simulink model "Boat_sim"  (Simulink 7.8)
settings: Solver=FixedStepDiscrete  StartTime=0.0  StopTime=1000  FixedStep=.01  RelTol=1e-3
InitFcn:
  | clear all
  | missions
  | common
  | physical_constants
  | simulation_constants
  | initial_values
  | l2plus
values from neighbouring files (symbols this model uses):
  InitialPoint = 0    [l2plus.m]
  IPStar = 0    [l2plus.m]
  MaxDwnPthStar = 1    [l2plus.m]
  OC2max = 49999    [simulation_constants.m]
  phi_0 = 0    [simulation_constants.m]
  switchDistance = 4    [l2plus.m]
  T_step = 0.01    [common.m]
  tanIntercept = tan( 45*pi/180 )    [l2plus.m]
  TStar = single(4.5)    [l2plus.m]
  Turn2Track = 0    [l2plus.m]
  wheelbase = 3.27    [physical_constants.m]
undefined symbols (not defined in the file or in its folder): DiscIntNeverNeededParam, Earth, figure8_waypoints, sampling_waypoints, test_waypoints, WGS84
libraries: simulink x21, uSimLib x21, instrumentlib x2, aerolibtransform2 x1, aerolibanimutils x1, simulink_need_slupdate x1
(part 2 of 2)

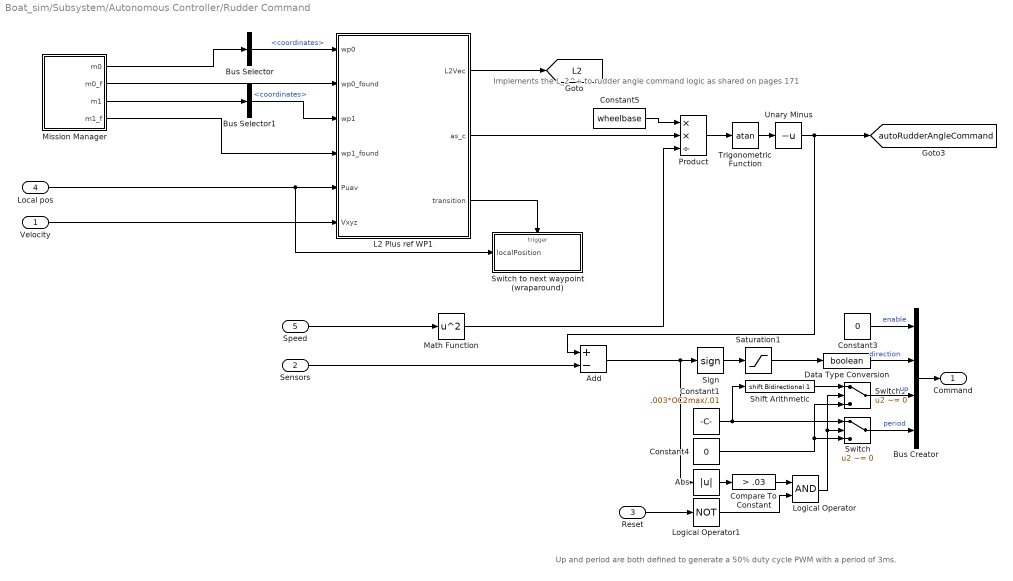
== system Boat_sim/Subsystem/Autonomous Controller/Rudder Command ==
  note: Up and period are both defined to generate a 50% duty cycle PWM with
      | a period of 3ms.
  note: Implements the L_2^+ to rudder angle command logic as shared on pages 171
  Velocity : Inport
  Sensors : Inport  Port=2
  Reset : Inport  Port=3
  Local pos : Inport  Port=4
  Speed : Inport  Port=5
  Abs : Abs
  Add : Sum  Inputs=+-
  Bus Creator : BusCreator
  Bus Selector : BusSelector  OutputSignals=coordinates
  Bus Selector1 : BusSelector  OutputSignals=coordinates
  Compare To Constant : simulink/Logic and Bit Operations/Compare To Constant  relop=>  const=.03  OutDataTypeStr=boolean
  Constant1 : Constant  Value=.003*OC2max/.01  OutDataTypeStr=uint16
  Constant3 : Constant  Value=0  OutDataTypeStr=boolean
  Constant4 : Constant  Value=0  OutDataTypeStr=uint16
  Constant5 : Constant  Value=wheelbase  OutDataTypeStr=boolean
  Data Type Conversion : DataTypeConversion  OutDataTypeStr=boolean  RndMeth=Simplest
  L2 Plus ref WP1 : MATLAB Function  TreatAsAtomicUnit=on
  Logical Operator : Logic  AllPortsSameDT=off  OutDataTypeStr=boolean
  Logical Operator1 : Logic  Operator=NOT  Inputs=1  AllPortsSameDT=off  OutDataTypeStr=boolean
  Math Function : Math  Operator=square  SaturateOnIntegerOverflow=on
  Mission Manager : Subsystem
  Product : Product  Inputs=**/  RndMeth=Zero
  Saturation1 : Saturate  UpperLimit=1  LowerLimit=0  OutDataTypeStr=Inherit: Inherit via back propagation
  Shift Arithmetic : ArithShift  BitShiftNumber=1
  Sign : Signum
  Switch : Switch  Criteria=u2 ~= 0
  Switch to next waypoint (wraparound) : Subsystem  TreatAsAtomicUnit=on
  Switch1 : Switch  Criteria=u2 ~= 0
  Trigonometric Function : Trigonometry  Operator=atan
  Unary Minus : UnaryMinus
  Command : Outport
  tag scope: L2=global, autoRudderAngleCommand=global
  wires:
  Bus Selector1/1 -> L2 Plus ref WP1/3(wp1)  "<coordinates>"
  Bus Selector/1 -> L2 Plus ref WP1/1(wp0)  "<coordinates>"
  Mission Manager/1(m0) -> Bus Selector/1
  Mission Manager/2(m0_f) -> L2 Plus ref WP1/2(wp0_found)
  L2 Plus ref WP1/3(transition) -> Switch to next waypoint (wraparound)/Trigger
  Mission Manager/4(m1_f) -> L2 Plus ref WP1/4(wp1_found)
  Mission Manager/3(m1) -> Bus Selector1/1
  Add/1 -> Abs/1, Sign/1
  Speed/1 -> Math Function/1
  Logical Operator1/1 -> Logical Operator/2
  Logical Operator/1 -> Switch1/2, Switch/2
  Compare To Constant/1 -> Logical Operator/1
  Local pos/1 -> Switch to next waypoint (wraparound)/1(localPosition), L2 Plus ref WP1/5(Puav)
  Reset/1 -> Logical Operator1/1
  Constant4/1 -> Switch1/3, Switch/3
  Switch1/1 -> Bus Creator/3  "up"
  Switch/1 -> Bus Creator/4  "period"
  Shift Arithmetic/1 -> Switch1/1
  Abs/1 -> Compare To Constant/1
  Constant1/1 -> Switch/1, Shift Arithmetic/1
  Constant3/1 -> Bus Creator/1  "enable"
  Velocity/1 -> L2 Plus ref WP1/6(Vxyz)
  L2 Plus ref WP1/1(L2Vec) -> [L2]
  Sign/1 -> Saturation1/1
  Saturation1/1 -> Data Type Conversion/1
  Bus Creator/1 -> Command/1
  Sensors/1 -> Add/2
  Data Type Conversion/1 -> Bus Creator/2  "direction"
  L2 Plus ref WP1/2(as_c) -> Product/2
  Constant5/1 -> Product/1
  Math Function/1 -> Product/3
  Product/1 -> Trigonometric Function/1
  Trigonometric Function/1 -> Unary Minus/1
  Unary Minus/1 -> Add/1, [autoRudderAngleCommand]

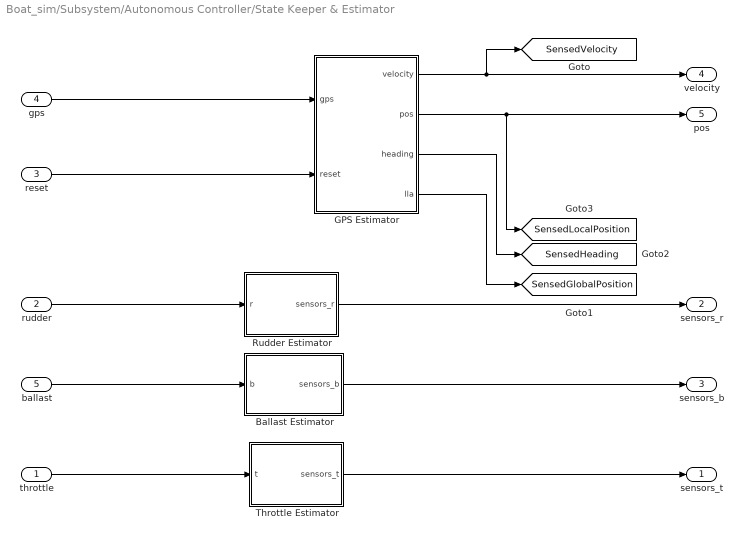
== system Boat_sim/Subsystem/Autonomous Controller/State Keeper & Estimator ==
  throttle : Inport
  rudder : Inport  Port=2
  reset : Inport  Port=3
  gps : Inport  Port=4
  ballast : Inport  Port=5
  Ballast Estimator : Subsystem
  GPS Estimator : Subsystem
  Rudder Estimator : Subsystem
  Throttle Estimator : Subsystem
  sensors_t : Outport
  sensors_r : Outport  Port=2
  sensors_b : Outport  Port=3
  velocity : Outport  Port=4
  pos : Outport  Port=5
  tag scope: SensedGlobalPosition=global, SensedHeading=global, SensedLocalPosition=global, SensedVelocity=global
  wires:
  Throttle Estimator/1(sensors_t) -> sensors_t/1
  Ballast Estimator/1(sensors_b) -> sensors_b/1
  Rudder Estimator/1(sensors_r) -> sensors_r/1
  GPS Estimator/4(lla) -> [SensedGlobalPosition]
  GPS Estimator/3(heading) -> [SensedHeading]
  GPS Estimator/2(pos) -> [SensedLocalPosition], pos/1
  gps/1 -> GPS Estimator/1(gps)
  GPS Estimator/1(velocity) -> [SensedVelocity], velocity/1
  reset/1 -> GPS Estimator/2(reset)
  throttle/1 -> Throttle Estimator/1(t)
  ballast/1 -> Ballast Estimator/1(b)
  rudder/1 -> Rudder Estimator/1(r)

== system Boat_sim/Subsystem/Autonomous Controller/Throttle Command ==
  sensors : Inport
  reset : Inport  Port=2
  Bus Creator : BusCreator
  Constant1 : Constant  Value=0  OutDataTypeStr=int16
  Constant5 : Constant  Value=1000  OutDataTypeStr=int16
  Mux Everything : Subsystem
  Switch : Switch  Criteria=u2 > Threshold
  Terminator : Terminator
  Trigger Events : Subsystem
  command : Outport
  tag scope: autoThrottleCommand=global
  wires:
  Constant5/1 -> Switch/3
  Constant1/1 -> Switch/1
  Switch/1 -> Trigger Events/1(RC Throttle), Mux Everything/4(Throttle), [autoThrottleCommand]
  Mux Everything/4(trig) -> Bus Creator/4  "trigger"
  Mux Everything/3(size) -> Bus Creator/3  "size"
  Mux Everything/2(data) -> Bus Creator/2  "data"
  Mux Everything/1(iden) -> Bus Creator/1  "identifier"
  reset/1 -> Switch/2, Trigger Events/2(Reset)
  Trigger Events/2(Disable) -> Mux Everything/2(disable)
  Trigger Events/3(Enable) -> Mux Everything/3(enable)
  Trigger Events/1(Change Speed) -> Mux Everything/1(speed)
  Bus Creator/1 -> command/1
  sensors/1 -> Terminator/1

== system Boat_sim/Subsystem/Log state data to workspace/Build HIL sentence ==
  data : Inport
  Bitwise Operator : simulink/Logic and Bit Operations/Bitwise Operator  logicop=XOR  UseBitMask=off  BitMask=bin2dec('11011001')  BitMaskRealWorld=Stored Integer
  Constant : Constant  Value=37  OutDataTypeStr=uint8
  Constant1 : Constant  Value=38  OutDataTypeStr=uint8
  Constant2 : Constant  Value=94  OutDataTypeStr=uint8
  Constant3 : Constant  Value=38  OutDataTypeStr=uint8
  Constant4 : Constant  Value=3  OutDataTypeStr=uint8
  Mux2 : Mux  Inputs=2
  Pack : MATLAB Function  TreatAsAtomicUnit=on
  sent : Outport
  wires:
  data/1 -> Mux2/2, Pack/4(d)
  Constant/1 -> Pack/1(a)
  Constant1/1 -> Pack/2(b)
  Pack/1(y) -> sent/1
  Constant4/1 -> Mux2/1, Pack/3(c)
  Constant2/1 -> Pack/5(e)
  Constant3/1 -> Pack/6(f)
  Bitwise Operator/1 -> Pack/7(g)
  Mux2/1 -> Bitwise Operator/1

== system Boat_sim/Plant/Actuator Dynamics/Subsystem/If Action Subsystem ==
  In1 : Inport
  Action Port : ActionPort  ActionType=then
  Bitwise Operator : simulink/Logic and Bit Operations/Bitwise Operator  logicop=OR  UseBitMask=off  NumInputPorts=2  BitMask=bin2dec('11011001')  BitMaskRealWorld=Stored Integer
  Data Store Write : DataStoreWrite  DataStoreName=throttle_speed
  Data Type Conversion : DataTypeConversion  OutDataTypeStr=uint16  ConvertRealWorld=Stored Integer (SI)
  Data Type Conversion2 : DataTypeConversion  OutDataTypeStr=double  LockScale=on
  Demux : Demux  Outputs=2
  Gain : Gain  Gain=1/1023
  Selector2 : Selector  InputPortWidth=6  IndexOptions=Index vector (dialog)  Indices=[4 3]  OutputSizes=1
  Shift Arithmetic : ArithShift  BitShiftNumber=-8
  wires:
  In1/1 -> Selector2/1
  Data Type Conversion2/1 -> Gain/1
  Gain/1 -> Data Store Write/1
  Selector2/1 -> Data Type Conversion/1
  Bitwise Operator/1 -> Data Type Conversion2/1
  Data Type Conversion/1 -> Demux/1
  Demux/1 -> Bitwise Operator/1
  Demux/2 -> Shift Arithmetic/1
  Shift Arithmetic/1 -> Bitwise Operator/2

== system Boat_sim/Subsystem/Autonomous Controller/Rudder Command/Mission Manager ==
  Data Type Conversion : DataTypeConversion  OutDataTypeStr=uint8
  GetCurrentMission : uSimLib/Mission Manager/GetCurrentMission  sampleTime=T_step
  GetMission : uSimLib/Mission Manager/GetMission  sampleTime=T_step
  If : If  IfExpression=u1 == 0
  If Action Subsystem : Subsystem  TreatAsAtomicUnit=on
  If Action Subsystem1 : Subsystem  TreatAsAtomicUnit=on
  Merge : Subsystem
  m0 : Outport
  m0_f : Outport  Port=2
  m1 : Outport  Port=3
  m1_f : Outport  Port=4
  wires:
  Data Type Conversion/1 -> GetMission/1
  Merge/2(found) -> m0_f/1
  Merge/1(mission) -> m0/1
  If Action Subsystem1/2(found) -> Merge/4(In4)
  If Action Subsystem/2(found) -> Merge/2(In3)
  If Action Subsystem1/1(mission) -> Merge/3(In2)
  If Action Subsystem/1(mission) -> Merge/1(In1)
  If/2 -> If Action Subsystem1/Action
  If/1 -> If Action Subsystem/Action
  GetMission/2 -> m1_f/1
  GetMission/1 -> m1/1
  GetCurrentMission/1 -> If/1, Data Type Conversion/1, If Action Subsystem1/1(i)

== system Boat_sim/Subsystem/Autonomous Controller/Rudder Command/Switch to next waypoint (wraparound) ==
  note: This block takes a triggering mission transition signal
      | and changes the current mission accordingly. It also
      | wraps the missions around if necessary from the last
      | mission to the first one.
  localPosition : Inport
  Trigger : TriggerPort
  Bias : Bias  Bias=1
  Data Type Conversion : DataTypeConversion  OutDataTypeStr=int8
  GetCurrentMission : uSimLib/Mission Manager/GetCurrentMission  sampleTime=-1
  GetMissionCount : uSimLib/Mission Manager/GetMissionCount  sampleTime=-1
  If : If  NumInputs=2  IfExpression=u1 < u2
  If Action Subsystem : Subsystem  TreatAsAtomicUnit=on
  If Action Subsystem1 : Subsystem  TreatAsAtomicUnit=on
  wires:
  localPosition/1 -> If Action Subsystem1/1(lPos)
  Data Type Conversion/1 -> If/2
  If/2 -> If Action Subsystem1/Action
  If/1 -> If Action Subsystem/Action
  Bias/1 -> If/1, If Action Subsystem/1(newIndex)
  GetMissionCount/1 -> Data Type Conversion/1
  GetCurrentMission/1 -> Bias/1

== system Boat_sim/Subsystem/Autonomous Controller/State Keeper & Estimator/Ballast Estimator ==
  b : Inport
  Bus Selector1 : BusSelector  OutputSignals=position
  sensors_b : Outport
  wires:
  Bus Selector1/1 -> sensors_b/1  "<position>"
  b/1 -> Bus Selector1/1

== system Boat_sim/Subsystem/Autonomous Controller/State Keeper & Estimator/GPS Estimator ==
  gps : Inport
  reset : Inport  Port=2
  Add : Sum
  Bus Selector1 : BusSelector  OutputSignals=newData
  Calculate local position from  GPS data : MATLAB Function  TreatAsAtomicUnit=on
  Discrete-Time Integrator4 : DiscreteIntegrator  ExternalReset=level  SampleTime=-1  ICPrevOutput=DiscIntNeverNeededParam  ICPrevScaledInput=DiscIntNeverNeededParam
  Subsystem : Subsystem
  velocity : Outport
  pos : Outport  Port=2
  heading : Outport  Port=3
  lla : Outport  Port=4
  tag scope: GpsOrigin=global, GpsOriginChanged=global
  wires:
  Calculate local position from  GPS data/4(refLLAChanged) -> [GpsOriginChanged]
  Calculate local position from  GPS data/3(refLLA) -> [GpsOrigin]
  Subsystem/1(velocity) -> Discrete-Time Integrator4/1, velocity/1
  Calculate local position from  GPS data/1(localPosition) -> Add/1
  Calculate local position from  GPS data/2(resetIntegrator) -> Discrete-Time Integrator4/2
  Bus Selector1/1 -> Calculate local position from  GPS data/2(newData)  "<newData>"
  Add/1 -> pos/1
  Discrete-Time Integrator4/1 -> Add/2
  Subsystem/3(pos) -> lla/1, Calculate local position from  GPS data/1(latLonAlt)
  gps/1 -> Bus Selector1/1, Subsystem/1(gps)
  Subsystem/2(heading) -> heading/1
  reset/1 -> Calculate local position from  GPS data/3(reset)

== system Boat_sim/Subsystem/Autonomous Controller/State Keeper & Estimator/Rudder Estimator ==
  r : Inport
  sensors_r : Outport
  wires:
  r/1 -> sensors_r/1

== system Boat_sim/Subsystem/Autonomous Controller/State Keeper & Estimator/Throttle Estimator ==
  t : Inport
  sensors_t : Outport
  wires:
  t/1 -> sensors_t/1

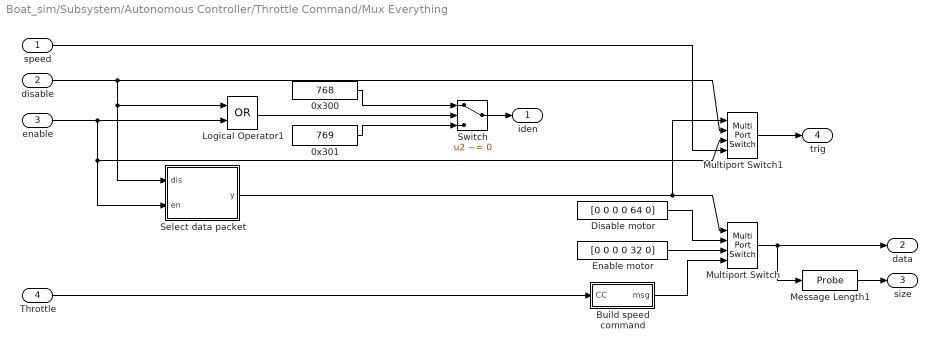
== system Boat_sim/Subsystem/Autonomous Controller/Throttle Command/Mux Everything ==
  speed : Inport
  disable : Inport  Port=2
  enable : Inport  Port=3
  Throttle : Inport  Port=4
  0x300 : Constant  Value=768  OutDataTypeStr=uint32
  0x301 : Constant  Value=769  OutDataTypeStr=uint32
  Build speed command : Subsystem
  Disable motor : Constant  Value=[0 0 0 0 64 0]  OutDataTypeStr=uint8
  Enable motor : Constant  Value=[0 0 0 0 32 0]  OutDataTypeStr=uint8
  Logical Operator1 : Logic  Operator=OR  AllPortsSameDT=off  OutDataTypeStr=boolean
  Message Length1 : Probe  ProbeSampleTime=off  ProbeComplexSignal=off  ProbeWidthDataType=uint8
  Multiport Switch : MultiPortSwitch  zeroidx=off
  Multiport Switch1 : MultiPortSwitch  zeroidx=off
  Select data packet : MATLAB Function  TreatAsAtomicUnit=on
  Switch : Switch  Criteria=u2 ~= 0
  iden : Outport
  data : Outport  Port=2
  size : Outport  Port=3
  trig : Outport  Port=4
  wires:
  Build speed command/1(msg) -> Multiport Switch/4
  speed/1 -> Multiport Switch1/4
  Multiport Switch1/1 -> trig/1
  Select data packet/1(y) -> Multiport Switch1/1, Multiport Switch/1
  Logical Operator1/1 -> Switch/2
  enable/1 -> Multiport Switch1/3, Select data packet/2(en), Logical Operator1/2
  disable/1 -> Multiport Switch1/2, Select data packet/1(dis), Logical Operator1/1
  Switch/1 -> iden/1
  0x301/1 -> Switch/3
  0x300/1 -> Switch/1
  Message Length1/1 -> size/1
  Multiport Switch/1 -> data/1, Message Length1/1
  Throttle/1 -> Build speed command/1(CC)
  Disable motor/1 -> Multiport Switch/2
  Enable motor/1 -> Multiport Switch/3

== system Boat_sim/Subsystem/Autonomous Controller/Throttle Command/Trigger Events ==
  RC Throttle : Inport
  Reset : Inport  Port=2
  Data Type Conversion1 : DataTypeConversion  OutDataTypeStr=boolean
  Data Type Conversion2 : DataTypeConversion  OutDataTypeStr=boolean
  Data Type Conversion3 : DataTypeConversion  OutDataTypeStr=boolean
  Detect Change : simulink/Logic and Bit Operations/Detect Change  vinit=0  InputProcessing=Inherited  OutDataTypeStr=uint8
  Detect Fall Nonpositive : simulink/Logic and Bit Operations/Detect Fall Nonpositive  vinit=0  InputProcessing=Inherited  OutDataTypeStr=uint8
  Detect Rise Positive : simulink/Logic and Bit Operations/Detect Rise Positive  vinit=0  InputProcessing=Inherited  OutDataTypeStr=uint8
  Shift Arithmetic : ArithShift  BitShiftNumber=2
  Weighted Moving Average : simulink_need_slupdate/Weighted Moving Average  mgainval=[.5 .5]  vinit=0.0  samptime=-1  OutDataTypeStr=Inherit: Inherit via back propagation  OutDataType=sfix(16)  OutScaling=2^-10  DoSatur=off  GainDataType=uint(16)  MatRadixGroup=Best Precision: Matrix-wise  GainScaling=2^-10
  Change Speed : Outport
  Disable : Outport  Port=2
  Enable : Outport  Port=3
  wires:
  Data Type Conversion1/1 -> Disable/1
  Data Type Conversion2/1 -> Enable/1
  Data Type Conversion3/1 -> Change Speed/1
  Detect Rise Positive/1 -> Data Type Conversion1/1
  Detect Fall Nonpositive/1 -> Data Type Conversion2/1
  Reset/1 -> Detect Rise Positive/1, Detect Fall Nonpositive/1
  Shift Arithmetic/1 -> Weighted Moving Average/1
  Weighted Moving Average/1 -> Detect Change/1
  Detect Change/1 -> Data Type Conversion3/1
  RC Throttle/1 -> Shift Arithmetic/1

== system Boat_sim/Subsystem/Autonomous Controller/Rudder Command/Mission Manager/If Action Subsystem ==
  Action Port : ActionPort  ActionType=then
  Constant : Constant  Value=true  OutDataTypeStr=boolean
  GetStartingPoint : uSimLib/Mission Manager/GetStartingPoint  sampleTime=-1
      link override Data Store Read: DataStoreElements=mList.startingPoint
  mission : Outport
  found : Outport  Port=2
  wires:
  Constant/1 -> found/1
  GetStartingPoint/1 -> mission/1

== system Boat_sim/Subsystem/Autonomous Controller/Rudder Command/Mission Manager/If Action Subsystem1 ==
  i : Inport
  Action Port : ActionPort  ActionType=else
  Bias : Bias  Bias=-1
  Data Type Conversion : DataTypeConversion  OutDataTypeStr=uint8
  GetMission : uSimLib/Mission Manager/GetMission  sampleTime=-1
      link override If Action Subsystem1/Selector: InputPortWidth=-1
  mission : Outport
  found : Outport  Port=2
  wires:
  Data Type Conversion/1 -> GetMission/1
  Bias/1 -> Data Type Conversion/1
  GetMission/2 -> found/1
  i/1 -> Bias/1
  GetMission/1 -> mission/1

== system Boat_sim/Subsystem/Autonomous Controller/Rudder Command/Mission Manager/Merge ==
  In1 : Inport
  In3 : Inport  Port=2
  In2 : Inport  Port=3
  In4 : Inport  Port=4
  Merge : Merge
  Merge1 : Merge
  mission : Outport
  found : Outport  Port=2
  wires:
  In4/1 -> Merge1/2
  Merge1/1 -> found/1
  In3/1 -> Merge1/1
  In2/1 -> Merge/2
  Merge/1 -> mission/1
  In1/1 -> Merge/1

== system Boat_sim/Subsystem/Autonomous Controller/Rudder Command/Switch to next waypoint (wraparound)/If Action Subsystem ==
  newIndex : Inport
  Action Port : ActionPort  ActionType=then
  Data Type Conversion : DataTypeConversion  OutDataTypeStr=uint8
  SetCurrentMission : uSimLib/Mission Manager/SetCurrentMission  sampleTime=-1
  wires:
  Data Type Conversion/1 -> SetCurrentMission/1
  newIndex/1 -> Data Type Conversion/1

== system Boat_sim/Subsystem/Autonomous Controller/Rudder Command/Switch to next waypoint (wraparound)/If Action Subsystem1 ==
  lPos : Inport
  Action Port : ActionPort  ActionType=else
  Bus Creator : BusCreator  Inputs='coordinates','refFrame','action','parameters','autocontinue'  OutDataTypeStr=Bus: Mission  NonVirtualBus=on
  Constant : Constant  Value=0  OutDataTypeStr=uint8
  Constant3 : Constant  Value=0  OutDataTypeStr=uint8
  Constant4 : Constant  Value=0  OutDataTypeStr=uint8
  Constant5 : Constant  Value=[0 0 0 0]  OutDataTypeStr=single
  Constant6 : Constant  Value=true  OutDataTypeStr=boolean
  SetCurrentMission : uSimLib/Mission Manager/SetCurrentMission  sampleTime=-1
  SetStartingPoint : uSimLib/Mission Manager/SetStartingPoint  sampleTime=-1
  wires:
  Constant6/1 -> Bus Creator/5  "autocontinue"
  Constant5/1 -> Bus Creator/4  "parameters"
  Constant4/1 -> Bus Creator/3  "action"
  Constant3/1 -> Bus Creator/2  "refFrame"
  lPos/1 -> Bus Creator/1  "coordinates"
  Bus Creator/1 -> SetStartingPoint/1
  Constant/1 -> SetCurrentMission/1

== system Boat_sim/Subsystem/Autonomous Controller/State Keeper & Estimator/GPS Estimator/Subsystem ==
  gps : Inport
  Bus Selector : BusSelector  OutputSignals=sog
  Bus Selector1 : BusSelector  OutputSignals=cog
  Bus Selector2 : BusSelector  OutputSignals=latitude,longitude,altitude
  Constant : Constant  Value=0  OutDataTypeStr=single
  Mux : Mux  Inputs=3
  Mux1 : Mux  Inputs=3
  Product : Product  OutDataTypeStr=single  RndMeth=Zero
  Product1 : Product  OutDataTypeStr=single  RndMeth=Zero
  Trigonometric Function : Trigonometry
  Trigonometric Function1 : Trigonometry  Operator=cos
  velocity : Outport
  heading : Outport  Port=2
  pos : Outport  Port=3
  wires:
  gps/1 -> Bus Selector/1, Bus Selector1/1, Bus Selector2/1
  Bus Selector1/1 -> heading/1, Trigonometric Function/1, Trigonometric Function1/1  "<cog>"
  Trigonometric Function/1 -> Product/2
  Trigonometric Function1/1 -> Product1/2
  Product1/1 -> Mux/1
  Product/1 -> Mux/2
  Constant/1 -> Mux/3
  Mux/1 -> velocity/1
  Bus Selector/1 -> Product1/1, Product/1  "<sog>"
  Bus Selector2/2 -> Mux1/2  "<longitude>"
  Bus Selector2/3 -> Mux1/3  "<altitude>"
  Mux1/1 -> pos/1
  Bus Selector2/1 -> Mux1/1  "<latitude>"

== system Boat_sim/Subsystem/Autonomous Controller/Throttle Command/Mux Everything/Build speed command ==
  CC : Inport
  Constant : Constant  OutDataTypeStr=uint8
  Constant1 : Constant  Value=0  OutDataTypeStr=uint8
  Constant2 : Constant  Value=0  OutDataTypeStr=uint8
  Constant3 : Constant  Value=5  OutDataTypeStr=uint8
  Mux : Mux  Inputs=5
  uint16 to uchar : Subsystem  AncestorBlock=uSimLib/Conversions/uint16 to uchar
  msg : Outport
  wires:
  uint16 to uchar/1(uchar) -> Mux/3
  Constant/1 -> Mux/1
  Constant3/1 -> Mux/2
  Mux/1 -> msg/1
  Constant1/1 -> Mux/4
  Constant2/1 -> Mux/5
  CC/1 -> uint16 to uchar/1(ushort)

== system Boat_sim/Subsystem/Autonomous Controller/Throttle Command/Mux Everything/Build speed command/uint16 to uchar ==
  ushort : Inport
  Data Type Conversion : DataTypeConversion  OutDataTypeStr=uint16  ConvertRealWorld=Stored Integer (SI)  RndMeth=Simplest
  Extract Bits1 : simulink/Logic and Bit Operations/Extract Bits  bitsToExtract=Upper half  numBits=8  bitIdxRange=[0 7]  outScalingMode=Treat bit field as an integer
  Extract Bits2 : simulink/Logic and Bit Operations/Extract Bits  bitsToExtract=Lower half  numBits=8  bitIdxRange=[0 7]  outScalingMode=Treat bit field as an integer
  Mux : Mux  Inputs=2
  uchar : Outport
  wires:
  Mux/1 -> uchar/1
  Extract Bits2/1 -> Mux/2
  Extract Bits1/1 -> Mux/1
  ushort/1 -> Data Type Conversion/1
  Data Type Conversion/1 -> Extract Bits1/1, Extract Bits2/1

== matlab function HIL Interface/Build HIL sentence/Pack ==
  data: a input double; y output double; b input double; c input double; d input double; e input double; f input double
function y = fcn(a, b, c, d, e, f)

y = zeros(40, 1, 'uint8');
y(1) = a;
y(2) = b;
y(3:37) = c;
y(38) = d;
y(39) = e;
y(40) = f;

== matlab function Plant/Get GPS/Embedded MATLAB Function1 ==
  data: cog output double; Vn input double; Ve input double
function cog = getCOG(Vn, Ve)
% This block supports an embeddable subset of the MATLAB language.
% See the help menu for details. 

cog = atan2(Vn,Ve);
if cog < 0;
    cog = cog + 2*pi;
end

== matlab function Subsystem/Autonomous Controller/State Keeper & Estimator/GPS Estimator/Calculate local position from GPS data ==
  data: latLonAlt input single size=[3 1]; localPosition output single; newData input boolean size=1; reset input boolean size=1; resetIntegrator output boolean size=1; refLLA output double; refLLAChanged output double
function [localPosition, resetIntegrator, refLLA, refLLAChanged] = estimateGPS(latLonAlt, newData, reset)
%#codegen

% This function watches an incoming stream of GPS data and outputs the
% current position in a local North-East-Down coordinate frame that is
% referenced from the 5th valid GPS fix that it received.

% INPUTS:
% latLonAlt - the latitude, longitude, and altitude of the vehicle from GPS
% in radians/meters.
% newData - A boolean signal specifying whether latLonAlt holds new data
% reset - A global reset boolean trigger.

% OUTPUTS:
% localPosition - The local position of the vehicle in meter within a
% North-East-Down coordinate frame. This reference frame is anchored at a
% specific GPS coordinate.
% resetIntegrator - Indicates that the velocity integrator, which is
% calculating position in between GPS fixes, should be reset.
% refLLA - The origin of the local frame in terms of global GPS coordinates in radians/meters.
% refLLAChanged - Whether the reference GPS position has changed in this
% timestep (boolean). Should only be changed when startingPosition is
% changed.

% Keep track of the origin of the local coordinate frame in
% startingPosition. Track the last valid GPS fix in lastKnownPosition.
% Track the state of this function within newDataCounter.
persistent startingPosition lastKnownPosition newDataCounter;

% Reset everything on first startup or when a global reset is triggered
if isempty(startingPosition) || reset
    startingPosition = zeros(3, 1, 'single');
end
if isempty(lastKnownPosition) || reset
    lastKnownPosition = zeros(3, 1, 'single');
end
if isempty(newDataCounter) || reset
    newDataCounter = uint8(0);
end

% Pass through the global reset to the velocity integrator
if reset
    resetIntegrator = true;
else
    resetIntegrator = false;
end

% Default the refLLAChanged signal to false.
refLLAChanged = false;

% Wait for 5 valid GPS inputs before latching a starting point
if newDataCounter < 5
    if newData && latLonAlt(1) ~= 0 && latLonAlt(2) ~= 0
        newDataCounter = newDataCounter + 1;
    end

    % We output all 0s while we're waiting
    localPosition = zeros(3, 1, 'single');
% If we have a valid GPS fix for the fifth catch, latch this as our origin
elseif newDataCounter == 5
    % Check that we have valid data before latching it.
    if newData && latLonAlt(1) ~= 0 && latLonAlt(2) ~= 0
        newDataCounter = newDataCounter + 1;
        startingPosition = latLonAlt;
        refLLAChanged = true;
    end
    
    % We output all 0s while we're waiting
    localPosition = zeros(3, 1, 'single');
% Finally just output the latched value
else
    % Latch a new position if one's been received. Also reset the integrator
    % for this timestep as we have a "truth" position now.
    if newData
        lastKnownPosition = latLonAlt;
        resetIntegrator = true;
    end
    
    % Calculate the difference between the starting position and the last
    % known position.
    localPosition = dg2lg(startingPosition, latLonAlt);
end

refLLA = startingPosition;

% Not certain how this works or where I got it from, but it translates two
% GPS coordinates in radians into a North-East-Down coordinates referenced
% from the u1 GPS location.
function out = dg2lg(u1, u2)

dlat = (u2(1) - u1(1));
dlon = (u2(2) - u1(2));
lat = u1(1);
h = u2(3);
a = 6378137;
e2 = 0.00669437999014;

v=a./sqrt(1-e2.*sin(lat).^2);
r=v.*(1-e2)./(1-e2.*sin(lat).^2);
dx=dlat.*(r+h);
dy=dlon.*cos(lat).*(v+h);

% Map into North-East-Down coordinates
out = [dx; dy; 0];

== matlab function HIL Interface/Parse HIL input/Embedded MATLAB Function ==
  data: successCount output double; failCount output double; in input uint8; out output uint8 size=27; new output double
function [successCount, failCount, out, new] = parseMessage(in)
    persistent actuatorMessage internalSuccessCount internalFailCount;
    
    if isempty(actuatorMessage)
        actuatorMessage = zeros(27, 1, 'uint8');
        internalSuccessCount = uint32(0);
        internalFailCount = uint32(0);
    end
    
    for i = 1:size(in,1)
        [new fail data] = buildAndCheckMessage(in(i));
        if new
            actuatorMessage = data;
            internalSuccessCount = internalSuccessCount + 1;
        elseif fail
            internalFailCount = internalFailCount + 1;
        end
    end
    successCount = internalSuccessCount;
    failCount = internalFailCount;
    out = actuatorMessage;
end

function [new fail data] = buildAndCheckMessage(characterIn)
%#eml

    persistent message messageIndex messageState actuatorData;

    if isempty(message)
        message = zeros(34, 1, 'uint8');
        messageIndex = uint8(0);
        messageState = uint8(0);
        actuatorData = zeros(27, 1, 'uint8');
    end

    % This contains the function's state of whether
    % it is currently building a message.
    % 0 - Awaiting header byte 0 (%)
    % 1 - Awaiting header byte 1 (&)
    % 2 - Building message
    % 3 - Awaiting header byte 0 (^)
    % 4 - Awaiting header byte 1 (&)
    % 5 - Reading checksum character

    new = false;
    fail = false;

    % We start recording a new message if we see the header
    if messageState == 0
        if characterIn == '%'
            message(1) = characterIn;
            messageIndex = uint8(2);
            messageState = uint8(1);
        else
            fail = true;
        end
    elseif messageState == 1
        % If we don't find the necessary ampersand we start over
        % waiting for a new sentence
        if characterIn == '&'
            message(2) = characterIn;
            messageIndex = messageIndex + 1;
            messageState = uint8(2);
        elseif characterIn ~= '%'
            messageIndex = uint8(1);
            messageState = uint8(0);
            fail = true;
        end
    elseif messageState == 2
        % Record every character that comes in now that we're building a sentence.
        % Only stop if we run out of room or an asterisk is found.
        message(messageIndex) = characterIn;
        messageIndex = messageIndex + 1;
        if messageIndex > 4 && message(4) < 249 && messageIndex == message(4) + 6
            if characterIn == '^'
                messageState = uint8(3);
            else
                messageState = uint8(0);
                messageIndex = uint8(1);
                fail = true;
            end
        elseif messageIndex == length(message) - 1
            % If we've filled up the buffer, ignore the entire message as we can't store it all
            messageIndex = uint8(1);
            messageState = uint8(0);
            fail = true;
        end
    elseif messageState == 3
        % If we don't find the necessary ampersand we continue
        % recording data as we haven't found the footer yet until
        % we've filled up the entire message (ends at 124 characters
        % as we need room for the 2 footer chars).
        message(messageIndex) = characterIn;
        messageIndex = messageIndex + 1;
        if characterIn == '&'
            messageState = uint8(4);
        elseif messageIndex == length(message)
            messageState = uint8(0);
            messageIndex = uint8(1);
            fail = true;
        end
    elseif messageState == 4
        % Record the checksum byte.
        message(messageIndex) = characterIn;

        % The checksum is now verified and if successful the message
        % is stored in the appropriate struct.
        checksumCalculated = uint8(0);
        for i=3:messageIndex-3
            checksumCalculated = bitxor(checksumCalculated, message(i));
        end

        if message(messageIndex) == checksumCalculated
            % If we've found an actuator message, update our local data store
            if message(3) == 2
                actuatorData = message(5:31);
                new = true;
            end
        else
            fail = true;
        end

        % We clear all state variables here regardless of success.
        messageIndex = uint8(1);
        messageState = uint8(0);
        message = zeros(34,1,'uint8');
    end

    data = actuatorData;
end

== matlab function Plant/Actuator Dynamics/Rudder angle rate change ==
  data: trigger input double; angle output double; direction input double; reset input double; resetToAngle input double
function angle = fcn(trigger, direction, reset, resetToAngle)
%#eml

% Keep a variable for tracking the rudder angle internally
persistent integratedAngle;
if isempty(integratedAngle)
    integratedAngle = single(0.0);
end

% Update the rudder angle given a reset
if reset
    integratedAngle = resetToAngle;
end

% If a trigger signal is received, increment the rudder 0.005rads in the
% proper direction. This is only done if the rudder hasn't reached the
% 45deg limit yet though.
if trigger
    if direction == 0 && integratedAngle > -0.785
        integratedAngle = integratedAngle - 0.0045;
    elseif direction == 1 && integratedAngle < 0.785
        integratedAngle = integratedAngle + 0.0045;
    end
end

% Finally output the calculated angle
angle = integratedAngle;

== matlab function Subsystem/Autonomous Controller/Rudder Command/L2 Plus ref WP1 ==
  data: wp0 input single size=3; wp0_found input boolean size=1; wp1 input single size=3; wp1_found input boolean size=1; L2Vec output single size=3; Puav input single size=3; Vxyz input single size=3; switchDistance parameter double size=1; tanIntercept parameter double size=1; MaxDwnPthStar parameter double size=1; Turn2Track parameter double size=1; InitialPoint parameter double size=1; IPStar parameter double size=1; TStar parameter double size=1; as_c output single size=1; transition output boolean size=1
function [L2Vec, as_c, transition] = L2PlusWP1(wp0, wp0_found, wp1, wp1_found, Puav, Vxyz, switchDistance, ...
    tanIntercept, MaxDwnPthStar,Turn2Track,...
    InitialPoint, IPStar, TStar)
%==============================
%     computes bank angle command for following a straight line
%     by creating an aim point that may be more than L2 away 
%     from the UAV. The aim point is (usually) farther along the path 
%     toward wp1 than the UAV, and the intercept
%     angle is less than or equal to a specified value. This limits the intercept
%     angle even when the UAV is within L2 of the path.
%     See L2PlusWP1.m for details
%
%         INPUTS   
%             T1      unit vector wp0-->wp1
%             N1      normal to T1
%             wp0     Mission bus with the from mission data in it
%             wp1     Mission bus with the to/current mission data in it
%             Puav    position of UAV
%             Vxyz    Inertial velocity
%             switchDistance distance from wp1 to switch to WP2
%
%         PARAMETERS
%             ISA_g   gravity
%             tanIntercept  tangent of intercept angle
%             MaxDwnPthStar L2 multiplier to determmine downpath aimpoint
%             Turn2Track    true to turn toward T1 instead of L2
%             InitialPoint  true if no line tracking at first--fly direct to some initial point
%             IPStar        L2 multiplier to determing distance of IP from first wp0
%             Tstar         was called L2Base, time constant of response
%             
%         OUTPUTS
%             L2Vec   L2 vector toward aim point
%             as_c    commanded lateral acceleration
%             transition A boolean of whether to transition or not to the next waypoint

    persistent IPActive;  %true if flying toward IP
    persistent IP; % location of initial point

    persistent direction; % Keep track of the direction for patrol mode
    if isempty(direction)
        direction = int8(1);
    end
    
    Pwp1 = single(zeros(3,1));
    Pe_y = single(0);
    Dist2wp1 = single(0);
    MinDownPath = single(0);
    Dist2WPSwitch = single(0);
    L2DownPath = single(0);
    L2ToT = single(zeros(3,1));
    L2Vec = single(zeros(3,1));
    IP1 = single([0; 0;-999]); %signal for no IP
    as_c = single(0);
    transition = false;
    
    Pne = [Puav(1); Puav(2); 0]; %horizontal position
    Vne = [Vxyz(1); Vxyz(2); 0]; % horizontal velocity
    Groundspeed = norm(Vne);
    L2 = single(TStar*Groundspeed);
    
    % If neither waypoint is valid then don't do anything
    if ~wp0_found || ~wp1_found
        return;
    % Otherwise if the first two waypoints are next to each other (as is
    % common if the origin is the first waypoint and the boat latches that
    % as its start value) then transition to the next waypoint.
    elseif norm(wp1 - wp0) < switchDistance
        transition = true;
        return;
    end
    
    % Calculate N1 and T1
    T1 = wp1 - wp0;
    T1 = T1/norm(T1);
    N1 = [-T1(2); T1(1); 0];
    
%     initialize the initial point
    if (isempty(IPActive))
        if (InitialPoint)
%             IP is set relative to the first "from" waypoint
            IPActive = -1;
            IP = [wp0(1); wp0(2); 0] - L2*IPStar*T1;
            
            if (norm(IP-Pne) < .001)
                IPActive = 0;
                IP = single([0; 0; -999]);
            end
        else
            IPActive = 0;
            IP = single([0; 0;-999]); %signal for no IP
        end
    end
    IP1 = IP;
    
    
    if (IPActive)
%         no line tracking, direct to IP
        L2Vec = L2*(IP - Pne)/norm(IP - Pne);
%         check to see if at the IP to terminate this mode
        if norm(IP - Pne) < .1*L2
            IPActive = 0;
        end
    else
         if (Pne(1) < 2)
             IP1 = IP1;
         end
%         IP not active, track WP lines
        Pwp1 = Pne - [wp1(1); wp1(2); 0]; % position of UAV relative to wp1
        Pe_y = single(Pwp1'*N1); % cross track error
        Dist2wp1 = -single(Pwp1'*T1); % distance to wp1

%         minimum down path distance for Aim Point intersection on T
%         is determined by the intercept angle but limited 
%         in case of very distant intecepts to MaxDwnPthStar*L2
        MinDownPath = single ( min( abs(Pe_y)/tanIntercept, MaxDwnPthStar*L2)); 
        Dist2WPSwitch = Dist2wp1 - switchDistance;
        if ( abs(Pe_y) > L2 )
    %             Make sure aimpoint is no closer to waypoint than calculated switch point.
            L2DownPath = MinDownPath;
        else
    %             within L2 of T and Dist2WPSwitch >= 0, but limit angle of L2 wrt T
            L2DownPath = (max(MinDownPath, (sqrt( L2^2 - Pe_y^2 ))));
        end
        
        if ( Dist2WPSwitch < 0 )
            transition = true;
        end
        
         % vector from Pwp1 to aim point on T1
         L2ToT = single(( Dist2wp1 - L2DownPath )*(-T1) - Pwp1);
         if (norm(L2ToT) < .001)
             L2Vec = L2*T1;
         else
            L2Vec = single(L2*( L2ToT/norm(L2ToT) )); % limit size to L2
         end
    %         L2Vec = L2ToT;
%         dummy statements
    end
    Zprod = single(Vxyz(1)*L2Vec(2) - Vxyz(2)*L2Vec(1)); %Z component of cross product
    sinEta = single(Zprod/(Groundspeed*L2));

    as_c = single(2*Groundspeed^2/(L2)*sinEta);

%         now override bank angle if heading in the wrong direction
    if ( Turn2Track && Dist2WPSwitch > 0 && ~IPActive ) 
%             turn to track not L2, gives min displacement from track
        if ( T1'*Vxyz < 0 )
            if ( Pe_y > 0 )
                as_c = single(99);
            else
                as_c = single(-99);
            end
        end
     else
%           turn toward L2, give min displacement toward wp0
        if ( L2Vec'*Vxyz < 0 )
            if ( sinEta < 0 )
                as_c = single(-99);
            else
                as_c = single(99);
            end
        end
    end
end

== matlab function Subsystem/Select current waypoint track ==
  data: reset output double; nextTrack input double; resetTrackNumber input double; test_waypoints parameter double; figure8_waypoints parameter double; sampling_waypoints parameter double
function reset  = selectTrack(nextTrack, resetTrackNumber, test_waypoints, figure8_waypoints, sampling_waypoints)
%#eml


% Initialize trackNumber.
% This variable is our state, which is the set of waypoints we're navigating
% between.
persistent trackNumber;
if isempty(trackNumber)
    trackNumber = uint8(1);
end

% Here is the logic for switching tracks. trackReset resets the trackNumber
% and nextTrack increments the track number
if resetTrackNumber
    trackNumber = uint8(1);
    reset = true;
elseif nextTrack
    trackNumber = trackNumber + uint8(1);
    if trackNumber > 3
        trackNumber = uint8(1);
    end
    reset = true;
else
    reset = false;
end

% 1 is for the test waypoints, 2 is for the figure eight, and 3 is
% for the data gathering waypoints.
% switch trackNumber
%     case 1
%         waypoints = test_waypoints;
%     case 2
%         waypoints = figure8_waypoints;
%     case 3
%         waypoints = sampling_waypoints;
%     otherwise
%         waypoints = zeros(size(test_waypoints), 'int32');
% end

== matlab function HIL Interface/Parse HIL input/Unpack sensor data ==
  data: u input uint8; rudderEnable output double; rudderDirection output double; rudderUp output double; rudderPeriod output double; ballastEnable output double; ballastDirection output double; throttleIdentifier output double; throttleData output double; throttleSize output double; throttleTrigger output double; timestamp output double; rudderAngle output double; sensorOverride output double
function [rudderEnable, rudderDirection, rudderUp, rudderPeriod, ballastEnable, ballastDirection, throttleIdentifier, throttleData, throttleSize, throttleTrigger, timestamp, rudderAngle, sensorOverride] = unpack(u)

rudderEnable = u(1);
rudderDirection = u(2);
rudderUp = typecast(u(3:4), 'uint16');
rudderPeriod = typecast(u(5:6), 'uint16');
ballastEnable = u(7);
ballastDirection = u(8);
throttleIdentifier = typecast(u(9:12), 'uint32');
throttleData = u(13:18);
throttleSize = u(19);
throttleTrigger = u(20);
timestamp = typecast(u(21:22), 'uint16');
rudderAngle = typecast(u(23:26), 'single');
sensorOverride = u(27);

== matlab function HIL Interface/Pack ==
  data: speed input double; lat input double; lon input double; alt input double; cog input double; sog input double; newData input double; y output double; rudderPosition input double; rudderStarboardLimit input double; rudderPortLimit input double; ballastPosition input double; ballastStarboardLimit input double; ballastPortLimit input double; timestamp input double
function y = u(speed, lat, lon, alt, cog, sog, newData, rudderPosition, rudderStarboardLimit, rudderPortLimit, ballastPosition, ballastStarboardLimit, ballastPortLimit, timestamp)

y = zeros(33, 1, 'uint8');
y(1:2) = typecast(speed, 'uint8');
y(3:6) = typecast(lat, 'uint8');
y(7:10) = typecast(lon, 'uint8');
y(11:14) = typecast(alt, 'uint8');
y(15:18) = typecast(cog, 'uint8');
y(19:22) = typecast(sog, 'uint8');
y(23) = newData;
y(24:25) = typecast(rudderPosition, 'uint8');
y(26) = rudderStarboardLimit;
y(27) = rudderPortLimit;
y(28:29) = typecast(ballastPosition, 'uint8');
y(30) = ballastStarboardLimit;
y(31) = ballastPortLimit;
y(32:33) = typecast(timestamp, 'uint8');

== matlab function Subsystem/Log state data to workspace/Build HIL sentence/Pack ==
  data: a input double; y output double; b input double; c input double; d input double; e input double; f input double; g input double
function y = fcn(a, b, c, d, e, f, g)
%#eml

y = uint8([a;b;c;d;e;f;g]);

== matlab function Subsystem/Log state data to workspace/Pack ==
  data: L2 input double; y output double; gPos input double; head input double; lPos input double; vel input double
function y = fcn(L2, gPos, head, lPos, vel)
%#eml

y = zeros(52, 1, 'uint8');
y(1:4) = packUint32BE(typecast(L2(1),'uint32'));
y(5:8) = packUint32BE(typecast(L2(2),'uint32'));
y(9:12) = packUint32BE(typecast(L2(3),'uint32'));
y(13:16) = packUint32BE(typecast(gPos(1),'uint32'));
y(17:20) = packUint32BE(typecast(gPos(2),'uint32'));
y(21:24) = packUint32BE(typecast(gPos(3),'uint32'));
y(25:28) = packUint32BE(typecast(head,'uint32'));
y(29:32) = packUint32BE(typecast(lPos(1),'uint32'));
y(33:36) = packUint32BE(typecast(lPos(2),'uint32'));
y(37:40) = packUint32BE(typecast(lPos(3),'uint32'));
y(41:44) = packUint32BE(typecast(vel(1),'uint32'));
y(45:48) = packUint32BE(typecast(vel(2),'uint32'));
y(49:52) = packUint32BE(typecast(vel(3),'uint32'));

function out = packUint32BE(in)
out = zeros(4, 1, 'uint8');
out(1) = uint8(bitand(bitshift(in,-24),hex2dec('FF')));
out(2) = uint8(bitand(bitshift(in,-16),hex2dec('FF')));
out(3) = uint8(bitand(bitshift(in,-8),hex2dec('FF')));
out(4) = uint8(bitand(in,hex2dec('FF')));

== matlab function HIL Interface/Parse HIL input/Embedded MATLAB Function2 ==
  data: u1 input double; y output double; u2 input double
function y = safeDiv(u1, u2)
%#eml

if u2 == 0
    y = u1;
else
    y = u1 / u2;
end

== matlab function Subsystem/Autonomous Controller/Throttle Command/Mux Everything/Select data packet ==
  data: y output double; dis input double; en input double
function y = fcn(dis, en)
% This block controls the switch selecting between enable, 
% disable, and speed commands. If disable and enable are
% both set high, disable overrides anything else.

y = uint8(3);
if dis == 1
    y = uint8(1);
elseif en == 1
    y = uint8(2);
end
